simulink model "controller_Arduino_soln"  (R2018a)
settings: Solver=FixedStepAuto  StartTime=0.0  StopTime=10.0  RelTol=1e-3  EnableMultiTasking=on
PreLoadFcn:
  | initParams;
values from neighbouring files (symbols this model uses):
  Ts = 0.01    [initParams.m]
libraries: arduinolib x3
settings Model: ExtModeTrigDuration=2  Creator=pmaier  LastModifiedBy=scastro
settings DataIOCC: LimitDataPoints=on  SaveFormat=Array
settings OptimizationCC: PassReuseOutputArgsAs=Individual arguments  MaxStackSize=64
settings DebuggingCC: UnderspecifiedInitializationDetection=Classic  MergeDetectMultiDrivingBlocksExec=none  SolverPrmCheckMsg=warning  ParameterTunabilityLossMsg=error  AllowSymbolicDim=off  StateNameClashWarn=warning  SFUnexpectedBacktrackingDiag=warning  SFNoUnconditionalDefaultTransitionDiag=warning  SFExecutionAtInitializationDiag=none
settings HardwareCC: ProdBitPerInt=16  ProdBitPerPointer=16  ProdBitPerSizeT=16  ProdBitPerPtrDiffT=16  ProdLargestAtomicFloat=None  ProdWordSize=8  ProdHWDeviceType=Atmel->AVR
settings ModelReferenceCC: PropagateSignalLabelsOutOfModel=off
settings SFSimCC: MATLABDynamicMemAlloc=off
settings RTWCC: SystemTargetFile=ert.tlc  HardwareBoard=Arduino Uno  TLCOptions=-aInlineSetEventsForThisBaseRateFcn=TLC_FALSE -aSuppressMultiTaskScheduler=TLC_FALSE -aRateBasedStepFcn=1  TemplateMakefile=ert_default_tmf  GenerateReport=on  Toolchain=Arduino AVR  BuildConfiguration=Faster Runs  IncludeHyperlinkInReport=on  LaunchReport=on  GenerateTraceInfo=on  GenerateTraceReport=on  GenerateTraceReportSl=on  GenerateTraceReportSf=on  GenerateTraceReportEml=on
settings CodeAppCC: ForceParamTrailComments=on  IgnoreCustomStorageClasses=off  OperatorAnnotations=on  SimulinkDataObjDesc=on  SFDataObjDesc=on  InsertBlockDesc=on
settings ERTTargetCC: SupportContinuousTime=on  SupportVariableSizeSignals=on
settings ConfigComp: CovMetricSettings=dw  CovHtmlReporting=on  CovSaveCumulativeToWorkspaceVar=on  CovSaveSingleToWorkspaceVar=on  CovExternalEMLEnable=off

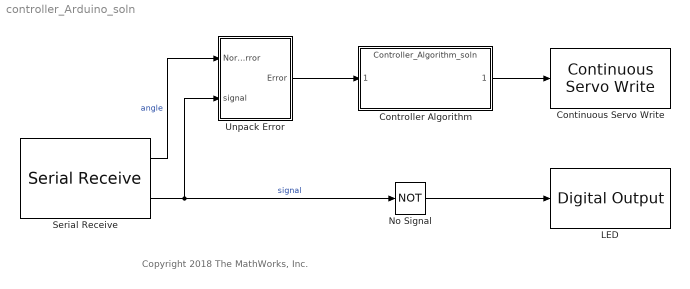
== system controller_Arduino_soln ==
  note: Copyright 2018 The MathWorks, Inc.
  Continuous Servo Write : arduinolib/Continuous Servo Write  pinNumber=9  blockPlatform=arduino
      settings: SourceProductName=Simulink Support Package for Arduino Hardware  SourceProductBaseCode=ARDUINO
  Controller Algorithm : ModelReference  ModelNameDialog=Controller_Algorithm_soln  SimulationMode=Normal  ModelReferenceVersion=1.21
  LED : arduinolib/Digital Output  pinNumber=13  blockPlatform=arduino
  No Signal : Logic  Operator=NOT  AllPortsSameDT=off  OutDataTypeStr=boolean
  Serial Receive : arduinolib/Serial Receive  isARMArch=off  portNumber=0  DataType=uint8  Datalength=1  SampleTime=Ts  showOutStatus=on  blockPlatform=arduino
      settings: SourceProductName=Simulink Support Package for Arduino Hardware  SourceProductBaseCode=ARDUINO
  Unpack Error : Subsystem
  wires:
  No Signal/1 -> LED/1
  Serial Receive/2 -> No Signal/1, Unpack Error/2(signal)  "signal"
  Serial Receive/1 -> Unpack Error/1(NormError)  "angle"
  Unpack Error/1(Error) -> Controller Algorithm/1
  Controller Algorithm/1 -> Continuous Servo Write/1

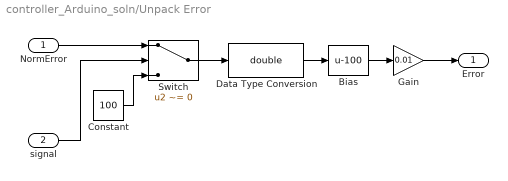
== system controller_Arduino_soln/Unpack Error ==
  NormError : Inport
  signal : Inport  Port=2
  Bias : Bias  Bias=-100
  Constant : Constant  Value=100
  Data Type Conversion : DataTypeConversion  OutDataTypeStr=double
  Gain : Gain  Gain=0.01
  Switch : Switch  Criteria=u2 ~= 0  Threshold=100
  Error : Outport
  wires:
  Switch/1 -> Data Type Conversion/1
  Bias/1 -> Gain/1
  Constant/1 -> Switch/3
  Gain/1 -> Error/1
  Data Type Conversion/1 -> Bias/1
  signal/1 -> Switch/2
  NormError/1 -> Switch/1
